simulink model "example_NMPC_BGLOSA_redTh_V500"  (R2022b)
settings: Solver=ode4  StartTime=0.0  StopTime=1000  FixedStep=0.1  RelTol=1e-3
PostLoadFcn:
  | , if any(exist('dsrtsu_mdlpostloadfcn', 'file') == [2, 3, 6]), try dsrtsu_mdlpostloadfcn('Execute', bdroot); catch fprintf('Error in PostLoadFcn (dsrtsu_mdlpostloadfcn) for model "%s":\n %s\n', bdroot, lasterr); end, end,
values from neighbouring files (symbols this model uses):
  N = 50    [NMPC_init.m]
  N_iter = 3    [NMPC_init.m]
  N_Jterms = length(Qx1)    [NMPC_init.m]
  NMPC_Wmat1 = [W1(1,:) W1(2,:) W1(3,:) W1(4,:) W1(5,:) W1(6,:) W1(7,:) W1(8,:)]    [NMPC_init.m]
  NMPC_WNmat1 = [WN1(1,:)]    [NMPC_init.m]
  t_dwell = 10    [NMPC_init.m]
  t_offset = 0    [NMPC_init.m]
  time_bag_sim = (0:1:round(time_bag(end))-1)'    [NMPC_init.m]
  tl_state_sim = zeros(round(time_bag(end))-1,size(tl_col,2))    [NMPC_init.m]
  Ts = 1    [NMPC_init.m]
  Vmax = 50    [NMPC_init.m]
  xInit = [0 2 0]    [NMPC_init.m]
libraries: simulink x1
settings Model: DSRTSU_INTERNAL_RTI_VER=450  DSRTSU_INTERNAL_RTI_TYPE=rti1401  DSRTSU_INTERNAL_RTIFPGA=40  Creator=d068515  LastModifiedBy=Daniele
settings DataIOCC: SaveFormat=StructureWithTime
settings OptimizationCC: BlockReduction=off  LifeSpan=inf
settings DebuggingCC: SFExecutionAtInitializationDiag=none  SFMachineParentedDataDiag=warning  ArithmeticOperatorsInVariantConditions=warning
settings HardwareCC: ProdBitPerSizeT=32  ProdBitPerPtrDiffT=32  ProdEndianess=BigEndian  ProdWordSize=32  ProdHWDeviceType=Generic->Custom  TargetIntDivRoundTo=Zero  TargetEndianess=BigEndian  TargetHWDeviceType=Generic->Custom
settings SFSimCC: CustomCodeUndefinedFunction=UseInterfaceOnly
settings RTWCC: Description=dSPACE DS1401 Hardware Platform  SystemTargetFile=rti1401.tlc  MakeCommand=make_rti  TemplateMakefile=rti1401.tmf
settings CodeAppCC: StateflowObjectComments=on
settings STFCustomTargetCC: ParMdlRefBuildCompliant=on  GRTInterface=on  SystemTargetFile=rti1401.tlc
settings GRTTargetCC: TargetLangStandard=C89/C90 (ANSI)  CompOptLevelCompliant=off  ConcurrentExecutionCompliant=off  CombineOutputUpdateFcns=off  MatFileLogging=off  CPPClassGenCompliant=off  GRTInterface=on  UseToolchainInfoCompliant=off  ExtModeMexFile=noextcomm

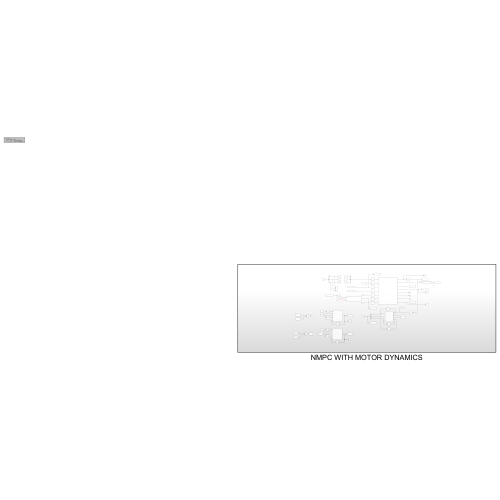
[thumbnail: Simulink's stored preview of the top-level diagram]
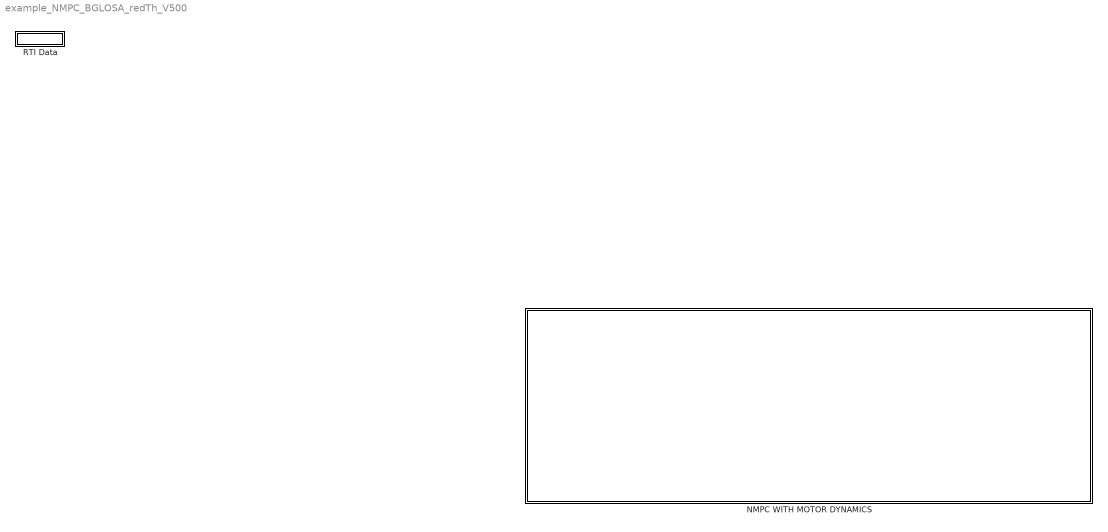
== system example_NMPC_BGLOSA_redTh_V500 ==
  NMPC WITH MOTOR DYNAMICS : Subsystem
  RTI Data : Subsystem  Tag=struct('RTIDataServer',struct('RTIDataServerVs','2','RTIModelDescription','struct(''main'',''TC_RAF_2014b'',''sub'','''',''isMp'',0)'))  LoadFcn="if exist('rtidc'), try,  rtidc('DataHostBlockClbLoad', gcbh); catch, disp(['Warning: ''LoadFcn'' for RTI Data block failed: ' lasterr]); end, end,"  mask(RTI_DATA_HOST){}
      mask help:
      | RTI Data Block.
      | This block is used by RTI to store internal model-dependent data.
      | Please keep this block on the root level of the model. Deleting this block will result in data loss.
      |
      | NEVER DELETE OR COPY THIS BLOCK!
      settings: CopyFcn="if exist('rtidc'), try,  rtidc('DataHostBlockClbCopy', gcbh); catch, disp(['Warning: ''CopyFcn'' for RTI Data block failed: ' lasterr]); end, end,"  DeleteFcn="if exist('rtidc'), try,  rtidc('DataHostBlockClbDelete', gcbh); catch, disp(['Warning: ''DeleteFcn'' for RTI Data block failed: ' lasterr]); end, end,"  ModelCloseFcn="if exist('rtidc'), try,  rtidc('DataHostBlockClbModelClose', gcbh); catch, disp(['Warning: ''ModelCloseFcn'' for RTI Data block failed: ' lasterr]); end, end,"  PreSaveFcn="if exist('rtidc'), try,  rtidc('DataHostBlockClbPreSave', gcbh); catch, disp(['Warning: ''PreSaveFcn'' for RTI Data block failed: ' lasterr]); end, end,"  PostSaveFcn="if exist('rtidc'), try,  rtidc('DataHostBlockClbPostSave', gcbh); catch, disp(['Warning: ''PostSaveFcn'' for RTI Data block failed: ' lasterr]); end, end,"  NameChangeFcn="if exist('rtidc'), try,  rtidc('DataHostBlockClbNameChange', gcbh); catch, disp(['Warning: ''NameChangeFcn'' for RTI Data block failed: ' lasterr]); end, end,"
      mask Help:
      | RTI Data Block.
      | This block is used by RTI to store internal model-dependent data.
      | Please keep this block on the root level of the model. Deleting this block will result in data loss.
      | 
      | NEVER DELETE OR COPY THIS BLOCK!
      mask Display:
      | text(0.5, 0.5, 'RTI Data', 'HorizontalAlignment', 'center');
      | plot([1 0]);

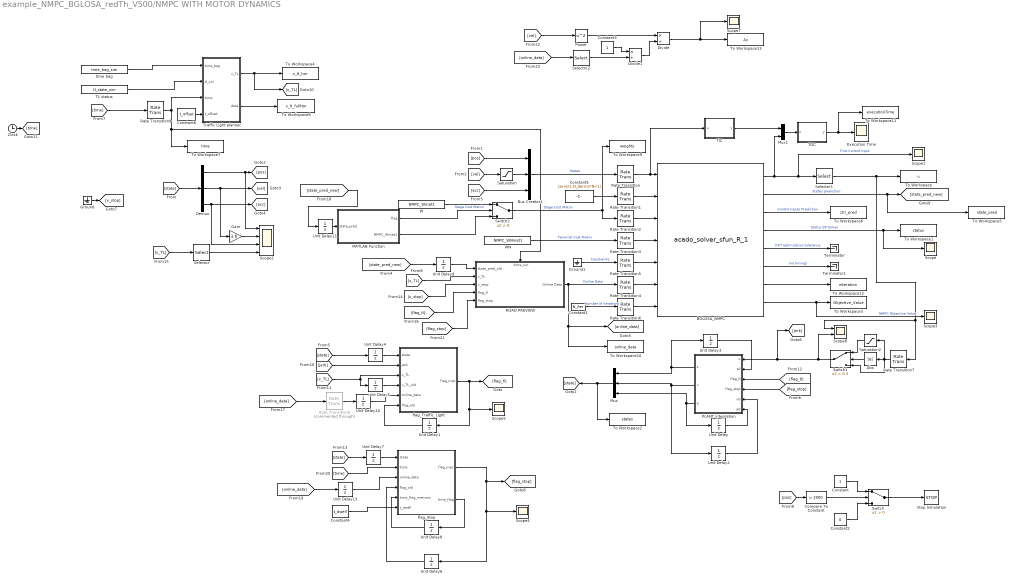
== system example_NMPC_BGLOSA_redTh_V500/NMPC WITH MOTOR DYNAMICS ==
  Abs : Abs  SaturateOnIntegerOverflow=off
  BGLOSA_NMPC : S-Function  FunctionName=acado_solver_sfun_R_1  Parameters=xInit, zInit, uInit, NMPC_Wmat1, NMPC_WNmat1, bValues  SFunctionDeploymentMode=off  EnableBusSupport=off  mask(Legacy Function){SFunctionSpec=acado_step(ACADOinput u1[1], ACADOoutput y1[1]), ShowSpec=on}
      mask prompts: ShowSpec "Display function specification"
      mask help:
      | This block allows you to call the legacy functions specified by the following Legacy Code Tool definition:
      | def.SFunctionName = 'acado_solver_sfun';
      | def.OutputFcnSpec = 'acado_step(ACADOinput u1[1], ACADOoutput y1[1])';
      | def.StartFcnSpec = 'acado_initialize( void )';
      | def.TerminateFcnSpec = 'acado_cleanup( void )';
      | def.HeaderFiles = {'acado_common.h', 'acado_solver_sfunction.h'};
      | def.SourceFiles = {'acado_solver.c', 'acado_integrator.c', 'acado_auxiliary_functions.c', 'acado_solver_sfunction.c', 'acado_qpoases_interface.cpp', 'qpoases/SRC/Bounds.cpp', 'qpoases/SRC/Constraints.cpp', 'qpoases/SRC/CyclingManager.cpp', 'qpoases/SRC/Indexlist.cpp', 'qpoases/SRC/MessageHandling.cpp', 'qpoases/SRC/QProblem.cpp', 'qpoases/SRC/QProblemB.cpp', 'qpoases/SRC/SubjectTo.cpp', 'qpoases/SRC/Utils.cpp', 'qpoases/SRC/EXTRAS/SolutionAnalysis.cpp'};
      | def.IncPaths = {'qpoases', 'qpoases/INCLUDE', 'qpoases/SRC'};
      | def.Options.language = 'C++';
      mask Help: <p>This block was generated automatically by the Legacy Code Tool. For detailed help on this tool, call<a href="matlab:legacy_code('help')"> legacy_code('help')</a>.</p>
      mask Callback ShowSpec:
      | if strcmp(get_param(gcbh, 'ShowSpec'), 'on')
      |   set_param(gcbh, 'MaskDisplay', sprintf('fprintf(''%s'');', get_param(gcbh, 'SFunctionSpec')));
      | else
      |   set_param(gcbh, 'MaskDisplay', sprintf('fprintf(''%s'');', get_param(gcbh, 'FunctionName')));
      | end
      mask Display: fprintf('acado_step(ACADOinput u1[1], ACADOoutput y1[1])');
  Bus Creator1 : BusCreator  Inputs=3
  Clock : Clock
  Compare To Constant : simulink/Logic and Bit Operations/Compare To Constant  relop=>  const=2000  OutDataTypeStr=boolean
  Constant : Constant
  Constant1 : Constant  Value=N_iter
  Constant2 : Constant  Value=0
  Constant3 : Constant
  Constant4 : Constant  Value=t_dwell
  Constant5 : Constant  Value=zeros(1,N_Jterms*N+1)
  Constant6 : Constant  Value=t_offset
  Demux : Demux  Outputs=3
  Divide : Product  Inputs=*/
  Divide1 : Product  Inputs=*/
  Execution Time : Scope
  Gain : Gain  Gain=3.6
  Ground : Ground
  Ground1 : Ground
  MATLAB Function : MATLAB Function  TreatAsAtomicUnit=on
  Mux : Mux  Inputs=3
  Mux1 : Mux  Inputs=2
  PLANT integration : MATLAB Function  TreatAsAtomicUnit=on
  Power : Math  Operator=square
  ROAD PREVIEW : Subsystem
      settings: PortSchema="{\"entries\":[{\"content\":{\"sides\":[{\"content\":{\"connectorIds\":[\"In1\",\"In2\",\"In3\",\"In4\",\"In5\"]},\"type\":\"ConnectorPlacement.EquallySpacedRectSide\",\"uuid\":\"89746bc5-bd2f-4e61-9556-28242176c46a\"},{\"content\":{\"connectorIds\":[\"Out1\"],\"side\":\"RIGHT\"},\"type\":\"ConnectorPlacement.EquallySpacedRectSide\",\"uuid\":\"fa5eae8e-eb55-42b4-8d8b-02c8b36cc91d\"},{\"content\":{\"connectorIds\":[\"In6\"],\"side\":\"TOP\"},\"type\":\"ConnectorPlacement.EquallySpacedRectSide\",\"uuid\":\"5942e98b-dfb5-4e56-acd3-edfb2315bb7f\"}]},\"type\":\"ConnectorPlacement.EquallySpacedConnector\",\"uuid\":\"ba8f73d0-227f-4198-ac0b-e11b2a073141\"}],\"packageUris\":[\"http://schema.mathworks.com/mf0/Connector/R2020b\"],\"version\":\"1.0\"}"
  Rate Transition : RateTransition  Deterministic=off  InitialCondition=xInit  OutPortSampleTime=Ts
  Rate Transition{1..6} (6 alike) : RateTransition  Deterministic=off  OutPortSampleTime=Ts
  Rate Transition7 : RateTransition  Deterministic=off  OutPortSampleTime=0.1
  Rate Transition8 : RateTransition  Commented=through  InitialCondition=zeros(1665,1)  OutPortSampleTime=Ts
  Rate Transition9 : RateTransition  OutPortSampleTime=Ts
  Saturation : Saturate  UpperLimit=50/3.6  LowerLimit=0
  Saturation2 : Saturate  UpperLimit=0.1  LowerLimit=-0.1
  Scope{,1,3..5,7} (6 alike) : Scope
  Scope2 : Scope  NumInputPorts=4
  Scope8 : Scope  NumInputPorts=2
  Selector : Selector  NumberOfDimensions=2  InputPortWidth=3  IndexOptions=Index vector (dialog),Select all  Indices=1,1  OutputSizes=1,1
  Selector1 : Selector  InputPortWidth=5  IndexOptions=Index vector (dialog)  Indices=[1]  OutputSizes=1
  Selector2 : Selector  NumberOfDimensions=2  InputPortWidth=3  IndexOptions=Index vector (dialog),Select all  Indices=27,1  OutputSizes=1,1
  Stop Simulation : Stop
  Switch : Switch  Criteria=u2 > Threshold  SaturateOnIntegerOverflow=off  InputSameDT=off
  Switch1 : Switch  Criteria=u2 > Threshold  Threshold=0.5  SaturateOnIntegerOverflow=off  InputSameDT=off
  Switch2 : Switch  Criteria=u2 > Threshold  SaturateOnIntegerOverflow=off  InputSameDT=off
  TIC : MATLAB Function  TreatAsAtomicUnit=on
  TL status : Constant  Value=tl_state_sim  OutDataTypeStr=double
  TOC : MATLAB Function  TreatAsAtomicUnit=on
  Terminator : Terminator
  Terminator1 : Terminator
  To Workspace : ToWorkspace  VariableName=u  SaveFormat=Structure With Time  SampleTime=-1
  To Workspace1 : ToWorkspace  VariableName=status  SaveFormat=Structure With Time  SampleTime=-1
  To Workspace10 : ToWorkspace  VariableName=online_data  SaveFormat=Structure With Time  SampleTime=-1
  To Workspace11 : ToWorkspace  VariableName=executionTime  SaveFormat=Structure With Time  SampleTime=-1
  To Workspace12 : ToWorkspace  VariableName=nIteration  SaveFormat=Structure With Time  SampleTime=-1
  To Workspace13 : ToWorkspace  VariableName=Ay  SaveFormat=Structure With Time  SampleTime=-1
  To Workspace2 : ToWorkspace  VariableName=states  SaveFormat=Structure With Time  SampleTime=-1
  To Workspace3 : ToWorkspace  VariableName=Objective_Value  SaveFormat=Structure With Time  SampleTime=-1
  To Workspace4 : ToWorkspace  VariableName=x_tl_hor  SaveFormat=Structure With Time  SampleTime=-1
  To Workspace5 : ToWorkspace  VariableName=state_pred  SaveFormat=Structure With Time  SampleTime=-1
  To Workspace6 : ToWorkspace  VariableName=ctrl_pred  SaveFormat=Structure With Time  SampleTime=-1
  To Workspace7 : ToWorkspace  VariableName=time  SaveFormat=Structure With Time  SampleTime=-1
  To Workspace8 : ToWorkspace  VariableName=x_tl_fullHor  SaveFormat=Structure With Time  SampleTime=-1
  To Workspace9 : ToWorkspace  VariableName=weights  SaveFormat=Structure With Time  SampleTime=-1
  Traffic Light planner : MATLAB Function  TreatAsAtomicUnit=on
  Unit Delay : UnitDelay  InitialCondition=xInit(3)  SampleTime=-1  HasFrameUpgradeWarning=on
  Unit Delay1 : UnitDelay  InitialCondition=zeros(1,12)  SampleTime=-1  HasFrameUpgradeWarning=on
  Unit Delay10 : UnitDelay  InitialCondition=zeros(25*(N+1),1)  SampleTime=-1  HasFrameUpgradeWarning=on
  Unit Delay11 : UnitDelay  InitialCondition=xInit.*ones(N+1,3)  SampleTime=-1  HasFrameUpgradeWarning=on
  Unit Delay13 : UnitDelay  InitialCondition=zeros(25*(N+1),1)  SampleTime=-1  HasFrameUpgradeWarning=on
  Unit Delay2 : UnitDelay  InitialCondition=xInit(2)  SampleTime=-1  HasFrameUpgradeWarning=on
  Unit Delay3 : UnitDelay  InitialCondition=xInit(1)  SampleTime=-1  HasFrameUpgradeWarning=on
  Unit Delay4 : UnitDelay  InitialCondition=xInit  SampleTime=-1  HasFrameUpgradeWarning=on
  Unit Delay5 : UnitDelay  InitialCondition=zeros(N+1,12)  SampleTime=-1  HasFrameUpgradeWarning=on
  Unit Delay6 : UnitDelay  InitialCondition=zeros(1,7)  SampleTime=-1  HasFrameUpgradeWarning=on
  Unit Delay7 : UnitDelay  InitialCondition=xInit  SampleTime=-1  HasFrameUpgradeWarning=on
  Unit Delay8 : UnitDelay  InitialCondition=zeros(1,7)  SampleTime=-1  HasFrameUpgradeWarning=on
  Unit Delay9 : UnitDelay  InitialCondition=xInit.*ones(N+1,3)  SampleTime=-1  HasFrameUpgradeWarning=on
  W : Constant  Value=NMPC_Wmat1  OutDataTypeStr=double
  "WN " : Constant  Value=NMPC_WNmat1  OutDataTypeStr=double
  flag_Stop : MATLAB Function  TreatAsAtomicUnit=on
  flag_Traffic_Light : MATLAB Function  TreatAsAtomicUnit=on
  time bag : Constant  Value=time_bag_sim  OutDataTypeStr=double
  wires:
  BGLOSA_NMPC/3 -> To Workspace6/1  "Control Inputs Prediction"
  BGLOSA_NMPC/4 -> To Workspace1/1, Scope/1  "Status QP Solver"
  Constant1/1 -> Rate Transition6/1  "Number of iterations"
  BGLOSA_NMPC/8 -> Scope3/1, To Workspace3/1  "NMPC Objective Value"
  Bus Creator1/1 -> Rate Transition/1  "States"
  BGLOSA_NMPC/1 -> Mux1/2, Scope1/1, Selector1/1  "First Control Input"
  BGLOSA_NMPC/5 -> Terminator/1  "KKT optimization tolerance"
  BGLOSA_NMPC/6 -> Terminator1/1  "(no timing)"
  Ground1/1 -> Rate Transition5/1  "Constraints"
  BGLOSA_NMPC/7 -> To Workspace12/1
  Rate Transition1/1 -> BGLOSA_NMPC/2
  Rate Transition2/1 -> BGLOSA_NMPC/3
  Rate Transition6/1 -> BGLOSA_NMPC/7
  Rate Transition3/1 -> BGLOSA_NMPC/4
  Rate Transition5/1 -> BGLOSA_NMPC/5
  Rate Transition4/1 -> BGLOSA_NMPC/6
  BGLOSA_NMPC/2 -> To Workspace5/1, [state_pred_new]  "States prediction"
  Constant5/1 -> Rate Transition1/1
  Demux/1 -> Scope2/1, [pos]
  Demux/2 -> [vel], Gain/1
  Demux/3 -> Scope2/3, [acc]
  PLANT integration/2(v) -> Mux/2, Unit Delay2/1
  PLANT integration/1(s) -> Unit Delay3/1, Mux/1
  PLANT integration/3(a) -> Mux/3, Unit Delay/1
  Unit Delay3/1 -> PLANT integration/2(s0)
  ROAD PREVIEW/1(Online Data) -> To Workspace10/1, [online_data], Rate Transition4/1  "Online Data"
  Switch2/1 -> Rate Transition2/1, To Workspace9/1  "Stage Cost Matrix"
  "WN "/1 -> Rate Transition3/1  "Terminal Cost Matrix"
  Selector1/1 -> Rate Transition7/1, Scope8/1, To Workspace/1
  Unit Delay/1 -> PLANT integration/6(a0)
  Unit Delay2/1 -> PLANT integration/5(v0)
  Mux/1 -> To Workspace2/1, [state]
  [state] -> Demux/1
  [pos] -> Bus Creator1/1
  [vel] -> Saturation/1
  [acc] -> Bus Creator1/3
  [state_pred_new] -> Unit Delay9/1
  [state] -> Unit Delay4/1
  [jerk] -> flag_Traffic_Light/2(jerk)
  [x_TL] -> ROAD PREVIEW/2(x_TL)
  [x_TL] -> Unit Delay5/1, flag_Traffic_Light/3(x_TL)
  flag_Traffic_Light/1(flag_mpc) -> [flag_tl], Scope5/1, Unit Delay1/1
  Unit Delay1/1 -> flag_Traffic_Light/6(flag_old)
  [flag_tl] -> PLANT integration/3(flag_tl)
  Unit Delay4/1 -> flag_Traffic_Light/1(state)
  Unit Delay5/1 -> flag_Traffic_Light/4(x_TL_old)
  [flag_stop] -> PLANT integration/4(flag_stop)
  Unit Delay7/1 -> flag_Stop/1(state)
  Unit Delay6/1 -> flag_Stop/4(flag_old)
  flag_Stop/1(flag_mpc) -> [flag_stop], Unit Delay6/1, Scope4/1
  [time] -> flag_Stop/2(time)
  [state] -> Unit Delay7/1
  [x_stop] -> ROAD PREVIEW/3(x_stop)
  Unit Delay9/1 -> ROAD PREVIEW/1(state_pred_old)
  time bag/1 -> Traffic Light planner/1(time_bag)
  TL status/1 -> Traffic Light planner/2(tl_col)
  Traffic Light planner/1(x_TL) -> [x_TL], To Workspace4/1
  Rate Transition9/1 -> ROAD PREVIEW/6(time_cur), To Workspace7/1, Traffic Light planner/3(time)
  [x_TL] -> Selector/1
  [flag_tl] -> ROAD PREVIEW/4(flag_tl)
  [online_data] -> Rate Transition8/1
  Unit Delay10/1 -> flag_Traffic_Light/5(online_data)
  Selector/1 -> Scope2/4
  Clock/1 -> [time]
  flag_Stop/2(time_flag) -> Unit Delay8/1
  Unit Delay8/1 -> flag_Stop/5(time_flag_memory)
  Ground/1 -> [x_stop]
  Saturation/1 -> Bus Creator1/2
  [pos] -> Compare To Constant/1
  Compare To Constant/1 -> Switch/2
  Constant/1 -> Switch/1
  Constant2/1 -> Switch/3
  Switch/1 -> Stop Simulation/1
  Rate Transition8/1 -> Unit Delay10/1
  [online_data] -> Unit Delay13/1
  Unit Delay13/1 -> flag_Stop/3(online_data)
  [flag_stop] -> ROAD PREVIEW/5(flag_stop)
  Switch1/1 -> Scope8/2, [jerk], PLANT integration/1(u)
  Rate Transition7/1 -> Saturation2/1, Switch1/3, Abs/1
  Abs/1 -> Switch1/2
  Saturation2/1 -> Switch1/1
  Gain/1 -> Scope2/2
  Power/1 -> Divide/1
  Divide1/1 -> Divide/2
  [vel] -> Power/1
  Constant3/1 -> Divide1/1
  [online_data] -> Selector2/1
  Selector2/1 -> Divide1/2
  Divide/1 -> Scope7/1, To Workspace13/1
  Constant4/1 -> flag_Stop/6(t_dwell)
  [time] -> Rate Transition9/1
  Traffic Light planner/2(data) -> To Workspace8/1
  Constant6/1 -> Traffic Light planner/4(t_offset)
  TOC/1(y) -> To Workspace11/1, Execution Time/1
  Rate Transition/1 -> TIC/1(u), BGLOSA_NMPC/1
  Mux1/1 -> TOC/1(u)
  TIC/1(y) -> Mux1/1
  W/1 -> Switch2/1  "Stage Cost Matrix"
  [state_pred_new] -> Unit Delay11/1
  Unit Delay11/1 -> MATLAB Function/1(state_pred)
  MATLAB Function/1(flag) -> Switch2/2
  MATLAB Function/2(NMPC_Wmat1) -> Switch2/3

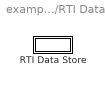
== system example_NMPC_BGLOSA_redTh_V500/RTI Data ==
  RTI Data Store : Subsystem  Tag="struct('private',struct('version',struct('dsVer',uint32(2),'dsVerCreation',uint32(2),'RTI',struct('ver','7.3','type','RTI1401')),'access',struct('type','Model','isPerm',1,'created',['23-Jan-2024 14:08:40'],'modified',['23-Jan-2024 15:26:34'],'location','')),'public',struct('main',struct('data',[]),'sub',struct('name',{{'TC_RAF_2014b'}},'data',{{struct('TH',struct('thTaskInfo',struct('taskType',{'TIMER','HWINT','TMRINT','SWINT','GLINT'},'tasksNumOf',{1,0,0,0,0},'srcIds',{{'TIMERA'},{},{},{},{}},'taskNames',{{['Timer Task 1']},{},{},{},{}})),'th_tc',struct('dataType','TASK','taskGroupId','','taskGroupList',{{}},'taskSchedulingPolicy','FCFS','taskType','TIMER','blkh',-1,'srcId','TIMERA','srcSgnName',['Timer A interrupt'],'srcCpuName','','taskName',['Timer Task 1  [0.01] s'],'taskNameDisplayExt','','smplTime',0.01,'smplTimeOffs',0,'hasFixedPriority',0,'priority',1,'hasFixedOvc',0,'ovcType',1,'ovcMax',1),'tc_th',struct('dataType','TASK','taskGroupId','','taskGroupList',{{}},'taskSchedulingPolicy','FCFS','taskType','TIMER','blkh',-1,'srcId','TIMERA','srcSgnName',['Timer A interrupt'],'srcCpuName','','taskName',['Timer Task 1  [0.01] s'],'taskNameDisplayExt','','smplTime',0.01,'smplTimeOffs',0,'hasFixedPriority',0,'priority',1,'hasFixedOvc',0,'ovcType',1,'ovcMax',1))}})))"  mask(RTI_DATA_STORE){}
      mask help:
      | RTI Data Store Block. This block is used by RTI to store internal model dependent data. Deleting this block will result in data loss.
      |
      | NEVER DELETE, COPY, OR MODIFY THIS BLOCK!
      mask Help:
      | RTI Data Store Block. This block is used by RTI to store internal model dependent data. Deleting this block will result in data loss.
      | 
      | NEVER DELETE, COPY, OR MODIFY THIS BLOCK!
      mask Display: text(0.5, 0.5, ' ', 'HorizontalAlignment', 'center');

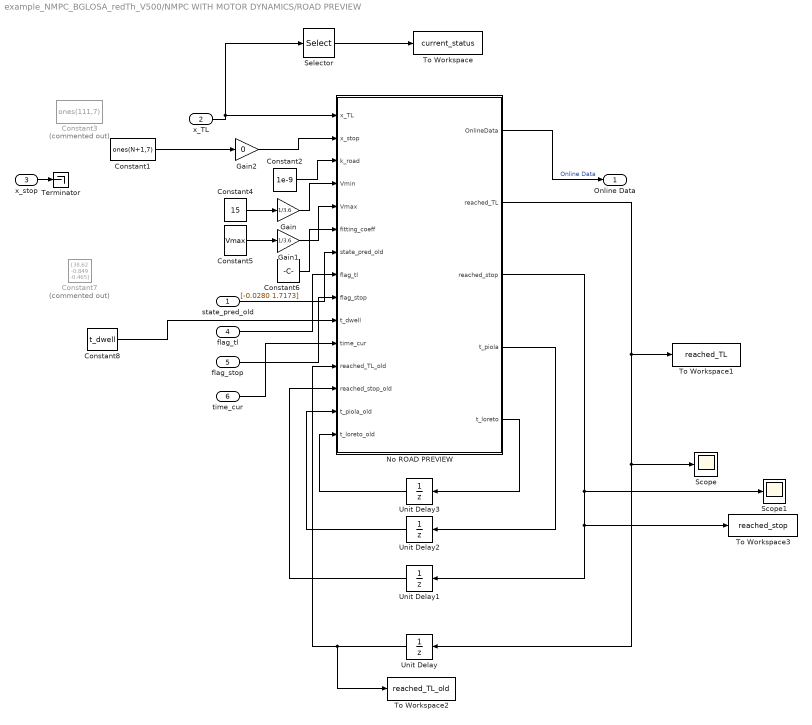
== system example_NMPC_BGLOSA_redTh_V500/NMPC WITH MOTOR DYNAMICS/ROAD PREVIEW ==
  state_pred_old : Inport
  x_TL : Inport  Port=2
  x_stop : Inport  Port=3
  flag_tl : Inport  Port=4
  flag_stop : Inport  Port=5
  time_cur : Inport  Port=6
  Constant1 : Constant  Value=ones(N+1,7)
  Constant2 : Constant  Value=1e-9
  Constant3 : Constant  Commented=on  Value=ones(111,7)
  Constant4 : Constant  Value=15
  Constant5 : Constant  Value=Vmax
  Constant6 : Constant  Value=[-0.0280 1.7173]
  Constant7 : Constant  Commented=on  Value=[38.62 -0.849 -0.465]
  Constant8 : Constant  Value=t_dwell
  Gain : Gain  Gain=1/3.6
  Gain1 : Gain  Gain=1/3.6
  Gain2 : Gain  Gain=0
  No ROAD PREVIEW : MATLAB Function  TreatAsAtomicUnit=on  SystemSampleTime=Ts
  Scope : Scope
  Scope1 : Scope
  Selector : Selector  NumberOfDimensions=2  InputPortWidth=3  IndexOptions=Index vector (dialog),Select all  Indices=1,1  OutputSizes=1,1
  Terminator : Terminator
  To Workspace : ToWorkspace  VariableName=current_status  SaveFormat=Structure With Time  SampleTime=-1
  To Workspace1 : ToWorkspace  VariableName=reached_TL  SaveFormat=Structure With Time  SampleTime=-1
  To Workspace2 : ToWorkspace  VariableName=reached_TL_old  SaveFormat=Structure With Time  SampleTime=-1
  To Workspace3 : ToWorkspace  VariableName=reached_stop  SaveFormat=Structure With Time  SampleTime=-1
  Unit Delay : UnitDelay  InitialCondition=zeros(1,11)  SampleTime=-1  HasFrameUpgradeWarning=on
  Unit Delay1 : UnitDelay  InitialCondition=zeros(1,7)  SampleTime=-1  HasFrameUpgradeWarning=on
  Unit Delay2 : UnitDelay  SampleTime=-1  HasFrameUpgradeWarning=on
  Unit Delay3 : UnitDelay  SampleTime=-1  HasFrameUpgradeWarning=on
  Online Data : Outport
  wires:
  No ROAD PREVIEW/1(OnlineData) -> Online Data/1  "Online Data"
  Constant2/1 -> No ROAD PREVIEW/3(k_road)
  Constant4/1 -> Gain/1
  Constant5/1 -> Gain1/1
  Constant6/1 -> No ROAD PREVIEW/6(fitting_coeff)
  Gain/1 -> No ROAD PREVIEW/4(Vmin)
  Gain1/1 -> No ROAD PREVIEW/5(Vmax)
  state_pred_old/1 -> No ROAD PREVIEW/7(state_pred_old)
  Constant1/1 -> Gain2/1
  Selector/1 -> To Workspace/1
  No ROAD PREVIEW/2(reached_TL) -> Unit Delay/1, Scope/1, To Workspace1/1
  Unit Delay/1 -> No ROAD PREVIEW/12(reached_TL_old), To Workspace2/1
  flag_tl/1 -> No ROAD PREVIEW/8(flag_tl)
  x_TL/1 -> Selector/1, No ROAD PREVIEW/1(x_TL)
  x_stop/1 -> Terminator/1
  flag_stop/1 -> No ROAD PREVIEW/9(flag_stop)
  No ROAD PREVIEW/3(reached_stop) -> To Workspace3/1, Unit Delay1/1, Scope1/1
  Unit Delay1/1 -> No ROAD PREVIEW/13(reached_stop_old)
  Gain2/1 -> No ROAD PREVIEW/2(x_stop)
  Constant8/1 -> No ROAD PREVIEW/10(t_dwell)
  No ROAD PREVIEW/4(t_piola) -> Unit Delay2/1
  No ROAD PREVIEW/5(t_loreto) -> Unit Delay3/1
  Unit Delay2/1 -> No ROAD PREVIEW/14(t_piola_old)
  Unit Delay3/1 -> No ROAD PREVIEW/15(t_loreto_old)
  time_cur/1 -> No ROAD PREVIEW/11(time_cur)

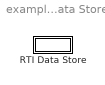
== system example_NMPC_BGLOSA_redTh_V500/RTI Data/RTI Data Store ==
  RTI Data Store : Subsystem  mask(RTI_DATA_STORE){}
      mask help:
      | RTI Data Store Block. This block is used by RTI to store internal model dependent data. Deleting this block will result in data loss.
      |
      | NEVER DELETE, COPY, OR MODIFY THIS BLOCK!
      mask Help:
      | RTI Data Store Block. This block is used by RTI to store internal model dependent data. Deleting this block will result in data loss.
      | 
      | NEVER DELETE, COPY, OR MODIFY THIS BLOCK!
      mask Display: text(0.5, 0.5, ' ', 'HorizontalAlignment', 'center');

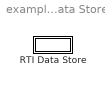
== system example_NMPC_BGLOSA_redTh_V500/RTI Data/RTI Data Store/RTI Data Store ==
  RTI Data Store : Subsystem  mask(RTI_DATA_STORE){}
      mask help:
      | RTI Data Store Block. This block is used by RTI to store internal model dependent data. Deleting this block will result in data loss.
      |
      | NEVER DELETE, COPY, OR MODIFY THIS BLOCK!
      mask Help:
      | RTI Data Store Block. This block is used by RTI to store internal model dependent data. Deleting this block will result in data loss.
      | 
      | NEVER DELETE, COPY, OR MODIFY THIS BLOCK!
      mask Display: text(0.5, 0.5, ' ', 'HorizontalAlignment', 'center');

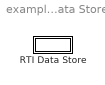
== system example_NMPC_BGLOSA_redTh_V500/RTI Data/RTI Data Store/RTI Data Store/RTI Data Store ==
  RTI Data Store : Subsystem  mask(RTI_DATA_STORE){}
      mask help:
      | RTI Data Store Block. This block is used by RTI to store internal model dependent data. Deleting this block will result in data loss.
      |
      | NEVER DELETE, COPY, OR MODIFY THIS BLOCK!
      mask Help:
      | RTI Data Store Block. This block is used by RTI to store internal model dependent data. Deleting this block will result in data loss.
      | 
      | NEVER DELETE, COPY, OR MODIFY THIS BLOCK!
      mask Display: text(0.5, 0.5, ' ', 'HorizontalAlignment', 'center');

== system example_NMPC_BGLOSA_redTh_V500/RTI Data/RTI Data Store/RTI Data Store/RTI Data Store/RTI Data Store ==

== matlab function example_NMPC_BGLOSA_redTh_V500/NMPC WITH MOTOR DYNAMICS/flag_Traffic_Light ==
  data: state input; jerk input; x_TL input; x_TL_old input; online_data input; flag_old input; flag_mpc output
function flag_mpc = fcn(state, jerk, x_TL, x_TL_old, online_data, flag_old)

s_TL = [45.5, 203.2, 384.2, 589.4, 773.6, 1004.2, 1225.3, 1419.7, 1507.8, 1739.0, 1823.0];
s_max = 5200;
N = 50;

flag_mpc = zeros(1,size(x_TL,2));
flag_old = flag_old';

for ii = 1:length(s_TL)

    if x_TL(1,ii) == x_TL_old(1,ii) % no status change for ii-th TL
        flag_old(1,ii) = flag_old(1,ii);
    else
        flag_old(1,ii) = 0;
    
    end
    
    if x_TL(1,ii) == 0 % red ii-th TL --> ii-th TL constraint active
        if state(2) < 0.1 && abs(s_TL(ii) - state(1)) < 0.5
            flag_mpc(ii) = 1;
        else 
            flag_mpc(ii) = 0;
        end
    else
        if abs(s_max - state(1)) < 0.5 && flag_old(1,ii) == 1 
            flag_mpc(ii) = 1;
        else
            flag_mpc(ii) = 0;
        end
    end

    if state(1) >= s_TL(ii) || sum(online_data(ii:22:end)) == N+1
        flag_mpc(ii) = 0;
    end

end

== matlab function example_NMPC_BGLOSA_redTh_V500/NMPC WITH MOTOR DYNAMICS/Traffic Light planner ==
  data: time_bag input; x_TL output; tl_col input; time input; data output; t_offset input
function [x_TL,data] = get_TL_data(time_bag, tl_col, time, t_offset)

time = time+round(t_offset);
N = 50;

x_TL = zeros(N+1,size(tl_col,2));
if time == 0
    t0 = 1;
else
    t0 = time_bag(time)+1;
end


for ii = 1:size(tl_col,2)
    if t0+N <= size(tl_col,1)
        x_TL(:,ii) = tl_col(t0:t0+N,ii);
    else
        x_TL(1:size(tl_col,1)-t0+1,ii) = tl_col(t0:end,ii);
    end
end

%%
data = zeros(N+1,size(tl_col,2));
time = time-round(t_offset);
if time == 0
    t0 = 1;
else
    t0 = time_bag(time)+1;
end


for ii = 1:size(tl_col,2)
    if t0+N <= size(tl_col,1)
        data(:,ii) = tl_col(t0:t0+N,ii);
    else
        data(1:size(tl_col,1)-t0+1,ii) = tl_col(t0:end,ii);
    end
end

== matlab function example_NMPC_BGLOSA_redTh_V500/NMPC WITH MOTOR DYNAMICS/MATLAB Function ==
  data: flag output; state_pred input; NMPC_Wmat1 output
function [flag, NMPC_Wmat1] = fcn(state_pred)

pos_hor = state_pred(:,1);

if pos_hor(1) > 1500 && pos_hor(1) < 1800
    flag = 0;
else
    flag = 1;
end

Qx1= [10 2 0.5 10 10000 10000 10000 10000];
W1 = diag(Qx1); 
NMPC_Wmat1=[W1(1,:) W1(2,:) W1(3,:) W1(4,:) W1(5,:) W1(6,:) W1(7,:) W1(8,:)];

== matlab function example_NMPC_BGLOSA_redTh_V500/NMPC WITH MOTOR DYNAMICS/TIC ==
  data: y output; u input
function y = fcn(u)
% The output y is of size 2x1.
%
% Zihao Liu 23/5/2020
% Last Change 23/5/2020

y = zeros(2,1);
t = tic; % During Code Gen, MATLAB returns a struct contains tv_sec and tv_nsec.
y(1) = t.tv_sec;
y(2) = t.tv_nsec;


end

== matlab function example_NMPC_BGLOSA_redTh_V500/NMPC WITH MOTOR DYNAMICS/TOC ==
  data: u input; y output
function y = fcn(u)
% Output y is a double scaler, in seconds.
%
%
% Zihao Liu 23/5/2020
% Last Change 23/5/2020


% Reconstruct the struct from tic.
t.tv_sec = u(1);
t.tv_nsec = u(2);
y = toc(t);

end

== matlab function example_NMPC_BGLOSA_redTh_V500/NMPC WITH MOTOR DYNAMICS/ROAD PREVIEW/No ROAD PREVIEW ==
  data: x_TL input; x_stop input; OnlineData output; k_road input; Vmin input; Vmax input; fitting_coeff input; state_pred_old input; flag_tl input; flag_stop input; t_dwell input; time_cur input; reached_TL_old input; reached_TL output; reached_stop_old input; reached_stop output; t_piola output; t_loreto output; t_piola_old input; t_loreto_old input
function [OnlineData, reached_TL, reached_stop, t_piola, t_loreto] = OnlineDataArray(x_TL, x_stop, k_road, Vmin, Vmax, fitting_coeff, state_pred_old, flag_tl, flag_stop, t_dwell, time_cur, reached_TL_old, reached_stop_old, t_piola_old, t_loreto_old )

s_TL = [45.5, 203.2, 384.2, 589.4, 773.6, 1004.2, 1225.3, 1419.7, 1507.8, 1739.0, 1823.0];
s_stop = [80, 447, 756, 1084, 1304, 1507, 1822]; 

N = size(x_TL,1)-1;
N_tl = length(s_TL);

pos_hor = state_pred_old(:,1);  % [m]
vel_hor = state_pred_old(:,2);  % [m/s]
% initialize online data variables
Ax_lim_mot = 1.15;     % [m/s^2]

x_TL1 = 1;  x_TL2 = 1;  x_TL3 = 1;  x_TL4 = 1;  
x_TL5 = 1;  x_TL6 = 1;  x_TL7 = 1;  x_TL8 = 1;
x_TL9 = 1;  x_TL10 = 1; x_TL11 = 1;

x_stop1 = x_stop(1);  x_stop2 = x_stop(2);  x_stop3 = x_stop(3);  x_stop4 = x_stop(4); x_stop5 = x_stop(5);  x_stop6 = x_stop(6);  x_stop7 = x_stop(7);
t_cur = time_cur; dt_schd = 180; s_st = 1e5; s_hor = 300; %s_hor = 240;

OnlineData = repmat([x_TL1; x_TL2; x_TL3; x_TL4; x_TL5; x_TL6; x_TL7; x_TL8; x_TL9; x_TL10; x_TL11; x_stop1; x_stop2; x_stop3; x_stop4; x_stop5; x_stop6; x_stop7; k_road; Vmin; Vmax; Ax_lim_mot; dt_schd; s_st; s_hor],N+1,1);


% a = fitting_coeff(1); b = fitting_coeff(2); c = fitting_coeff(3);
m = fitting_coeff(1); q = fitting_coeff(2);
v = vel_hor.*3.6;       % [km/h]

% build constraint on max acc. as a function of vehicle speed (motor limit)
for kk = 1:length(v)
    if v(kk) > 20
        Ax_lim = m*v(kk) + q;   % [m/s^2]
        OnlineData(22 + (kk-1)*25) = Ax_lim;
    end
end

% provide Bus Stop onlide data throughout the prediction horizon
reached_stop = reached_stop_old;
N_stops = length(s_stop);
for jj = 1:N_stops
    if pos_hor(1) >= s_stop(jj)
        OnlineData(N_tl + jj:25:end) = 1;
        continue
    end
    if reached_stop(jj) == 0 && abs(pos_hor(1) - s_stop(jj)) < 0.5 && vel_hor(1) < 0.01
        reached_stop(jj) = 1;
    else
        if reached_stop(jj) <= t_dwell && abs(pos_hor(1) - s_stop(jj)) < 0.5 && vel_hor(1) < 0.01
            reached_stop(jj) = reached_stop(jj) + 1;
        else
            reached_stop(jj) = reached_stop(jj);
        end
    end
    if reached_stop(jj) > t_dwell
        OnlineData(N_tl + jj:25:end) = 1;
    else
        OnlineData(N_tl + jj:25:end) = 0;
    end
    
end

map_road = coder.load('PL_jrl_chs.mat');


% provide road-curvature data throughout the prediction horizon
k_road_real = ones(N+1,1);
for kk = 1:N+1
    s = pos_hor(kk);
    [~,~,~,C_c,~,~] = Map_loc(map_road.map_road,s);
    OnlineData(N_tl+N_stops+1 + 25*(kk-1)) = abs(C_c);
    k_road_real(kk) = abs(C_c);
end


% provide online data throughout the prediction horizon for schedule adherance

if pos_hor(1) > s_stop(1) 
    t_piola = t_piola_old;
else
    t_piola = time_cur;
end
if pos_hor(1) > s_stop(3) 
    t_loreto = t_loreto_old;
else
    t_loreto = time_cur;
end

if pos_hor(1) > 1510
    aaa = 1;
end

for kk = 1:N+1
    if pos_hor(kk) <= s_stop(3)
        t_target = 180-10;
        t_prev_stop = t_piola;
    else
        t_target = 480-10;
        t_prev_stop = t_loreto;
    end
    OnlineData(23 + 25*(kk-1)) = t_target - (t_cur - t_prev_stop + (kk-1));
    if pos_hor(kk) <= s_stop(1)
        OnlineData(24 + 25*(kk-1)) = 1e5;
    elseif pos_hor(kk) > s_stop(1) && pos_hor(kk) <= s_stop(3)
%         t_target = 180;
%         OnlineData(23 + 25*(kk-1)) = t_target - (t_cur - t_piola + (kk-1));
        OnlineData(24 + 25*(kk-1)) = s_stop(3);
    elseif pos_hor(kk) > s_stop(3) && pos_hor(kk) <= s_stop(end)
%         t_target = 480;
%         OnlineData(23 + 25*(kk-1)) = t_target - (t_cur - t_loreto + (kk-1));
        OnlineData(24 + 25*(kk-1)) = s_stop(end);
    else
        OnlineData(24 + 25*(kk-1)) = 1e5;
    end
end

% provide TL onlide data throughout the prediction horizon
reached_TL = reached_TL_old;
kk_turn_red = 1;
kk_turn_green = 1;

for ii = 1:N_tl
    if pos_hor(1) >= s_TL(ii)
        OnlineData(ii:25:end) = 1;
        continue
    end
%     OnlineData(ii) = x_TL(1,ii);
    for kk = 2:N+1

%         OnlineData(ii + 15*(kk-1)) = x_TL(kk,ii); 
        if pos_hor(1) > 1510 %&& kk == 30
            aaa = 1;
        end
        if pos_hor(1) > 1600 %&& kk == 30
            aaa = 1;
        end
        if pos_hor(1) > 1650 %&& kk == 30
            aaa = 1;
        end
        if pos_hor(1) > 1700 %&& kk == 30
            aaa = 1;
        end
        
        i_pass_tl = find(pos_hor>s_TL(ii),1,"first");
        if (isempty(i_pass_tl) && abs(s_TL(ii) - pos_hor(1)) > 5) || (x_TL(1,ii)==1 && reached_TL(ii) == 1)
            OnlineData(ii + 25*(kk-1):25:end) = 1;
        elseif isempty(i_pass_tl) && abs(s_TL(ii) - pos_hor(1)) <= 5
            OnlineData(ii + 25*(kk-1):25:end) = 0;
        else
            if i_pass_tl > 1
                if x_TL(1,ii) == 0
                    kk_turn_green = find(x_TL(:,ii)==1,1,"first")+1;
                    if kk <= kk_turn_green
                        OnlineData(ii + 25*(kk-1)) = 0;
                    elseif isempty(kk_turn_green)
                        OnlineData(ii + 25*(kk-1)) = 0;
                    end
%                     is_green = find(x_TL(:,ii)==1);
%                     if not(isempty(is_green))
%                         kk_turn_red = is_green(end)+1;
%                         if i_pass_tl >= kk_turn_red
%                             
% %                             OnlineData(ii + 25*(kk_turn_red-1):25:end) = 0;
%                         end
%                     end
                else
                    if x_TL(i_pass_tl-1,ii) == 1 %&& x_TL(i_pass_tl,ii) == 1
                        OnlineData(ii:25:end) = 1;
                    else
                        kk_turn_red = min(find(x_TL(:,ii)==0));
                        if not(isempty(kk_turn_red))
                            if isempty(find(x_TL(kk_turn_red:end,ii)==1))
                                OnlineData(ii + 25*(kk-1)) = 0;
                            else
                                kk_turn_green = min(find(x_TL(kk_turn_red:end,ii)==1)) + kk_turn_red - 1;
                                if kk <= kk_turn_green || kk > kk_turn_red
                                    OnlineData(ii + 25*(kk-1)) = 0;
                                end
                            end
                        else
                            OnlineData(ii + 25*(i_pass_tl-1)) = 0;
                            OnlineData(ii + 25*(i_pass_tl-1 -1)) = 0;
                        end
                    end
                end
            else
                OnlineData(ii + 25*(kk-1):25:end) = 1;
            end

            if (abs(pos_hor(1) - s_TL(ii)) < 0.5 && vel_hor(1) < 0.01) || reached_TL(ii) == 1        % reached ii-th TL
                reached_TL(ii) = 1;
                if x_TL(1,ii) == 1
                    OnlineData(ii:25:end) = 1;
                else
                    OnlineData(ii + 25*(kk-1)) = x_TL(kk,ii);
                end
            else
                reached_TL(ii) = 0;
            end
            
%             if reached_TL(ii) == 1 && x_TL(1,ii) == 1
%                 OnlineData(ii:15:end) = 1;
%             else
%                 OnlineData(ii + 15*(kk-1)) = x_TL(kk,ii); 
%             end  
        end
    end
    if pos_hor(1) > s_TL(ii)+10
        OnlineData(ii:25:end) = 1;
    end
end


aaa = 1;

== matlab function example_NMPC_BGLOSA_redTh_V500/NMPC WITH MOTOR DYNAMICS/flag_Stop ==
  data: state input; time input; online_data input; flag_old input; time_flag_memory input; flag_mpc output; time_flag output; t_dwell input
function [flag_mpc, time_flag] = fcn(state, time, online_data, flag_old, time_flag_memory, t_dwell)

s_stop = [80, 447, 756, 1084, 1304, 1507, 1822];
s_max = 5200;
N_stop = length(s_stop);

flag_mpc = zeros(1,N_stop);
flag_old = flag_old';
time_flag = time_flag_memory';

for jj = 1:length(s_stop)
%     if time_flag(1,jj) == 0 && state(2) < 0.01 && abs(s_stop(jj) - state(1)) < 1 
%         flag_mpc(1,jj) = 1;
%         time_flag(1,jj) = time;
%     else
%         flag_old(1,jj) = flag_old(1,jj);
%         time_flag(1,jj) = time_flag_memory(jj);
%     end
% 
%     if time_flag(1,jj) - time > 10 || state(1) < s_stop(jj)
%         flag_mpc(jj) = 0;
%     else 
%         flag_mpc(jj) = 1;
%     end
    
    if state(2) < 0.01 && abs(s_stop(jj) - state(1)) < 0.5 
        if time_flag_memory(jj) == 0 
            time_flag(1,jj) = time;     % dwell initial time
            flag_mpc(1,jj) = 1;
        else
            if time - time_flag_memory(jj) > t_dwell
                flag_mpc(1,jj) = 0;
            else
                flag_mpc(1,jj) = 1;
            end
        end     
    else
        flag_mpc(1,jj) = 0;
    end

end

== matlab function example_NMPC_BGLOSA_redTh_V500/NMPC WITH MOTOR DYNAMICS/PLANT integration ==
  data: s output; v output; a output; u input; s0 input; flag_tl input; flag_stop input; v0 input; a0 input
function [s, v, a]= plant_integrator(u, s0, flag_tl, flag_stop, v0, a0)

dt = 0.1;
s_TL = [45.5, 203.2, 384.2, 589.4, 773.6, 1004.2, 1225.3, 1419.7, 1507.8, 1739.0, 1823.0];
s_stop = [80, 447, 756, 1084, 1304, 1507, 1822]; 

next_tl = find(s_TL>s0);
next_stop = find(s_stop>s0);

% if isempty(next_tl)
%     a = a0 + u*dt;
%     v = v0 + a*dt;
%     s = s0 + v*dt;
% else
%     i_next_tl = next_tl(1);
%     if flag_tl(i_next_tl) == 1 %|| flag_stop == 1
%         a = 0;
%         v = 0;
%         s = s0;
%     else
%         a = a0 + u*dt;
%         v = v0 + a*dt;
%         s = s0 + v*dt;
%     end
% end



if isempty(next_stop)       % no more stops ahead
    if isempty(next_tl)     % no more TL ahead
        a = a0 + u*dt;
        v = v0 + a*dt;
        s = s0 + v*dt;
    else                    % no stops ahead but at least one TL remaining
        i_next_tl = next_tl(1);
        if flag_tl(i_next_tl) == 1  % TL red --> ignore control action
            a = 0;
            v = 0;
            s = s0;
        else                        % TL green --> keep on integrating
            a = a0 + u*dt;
            v = v0 + a*dt;
            s = s0 + v*dt;
        end
    end
else                        % at least one stop remaining
    if isempty(next_tl)     % no more TL ahead
        a = a0 + u*dt;
        v = v0 + a*dt;
        s = s0 + v*dt;
    else                    % at least one TL and one stop remaining
        i_next_tl = next_tl(1);
        j_next_stop = next_stop(1);
%         if s0 > 200% && v0 == 0 && flag_stop(1) == 0
%             aaa = 1;
%         end
        if s_stop(j_next_stop) < s_TL(i_next_tl)
            if flag_stop(j_next_stop) == 1 && s_stop(j_next_stop) - s0 < 1
                a = 0;
                v = 0;
                s = s0;
            else
                a = a0 + u*dt;
                v = v0 + a*dt;
                s = s0 + v*dt;
            end
        else
            if flag_tl(i_next_tl) == 1 && s_TL(i_next_tl) - s0 < 1
                a = 0;
                v = 0;
                s = s0;
            else
                a = a0 + u*dt;
                v = v0 + a*dt;
                s = s0 + v*dt;
            end
        end
    end
end
